simulink model "FeedbackLin"  (R2016a)
settings: Solver=ode45  StartTime=0.0  StopTime=2*Tpasso  FixedStep=1e-4  RelTol=1e-5
values from neighbouring files (symbols this model uses):
  Bm = 1e-4    (= 0.0001)    [runTests.m]
  cm = [c1; c2; c3; c4; c5]    [runTests.m]
  Cphi = 1    [runTests.m]
  cr = [c1; c2; c3; c4; c5]    [runTests.m]
  dQ0 = [dQ10; dQ20; dQ30; dQ40; dQ50]    [runNoErrorNoNoiseNoIncNoFext.m]    (also in runTests.m = zeros(5,1))
  gait = 1    [runTests.m]
  gm = g    (= 9.81)    [runTests.m]
  gr = g    (= 9.81)    [runTests.m]
  Im = [I1; I2; I3; I4; I5]    [runTests.m]
  Ir = [I1; I2; I3; I4; I5]    [runTests.m]
  Jm = 5e-3    (= 0.005)    [runTests.m]
  Kt = 0.1    [runTests.m]
  La = 1e-3    (= 0.001)    [runTests.m]
  LambdaFL = [150; 150; 150; 150]    [runTests.m]
  lm = [l1; l2; l3; l4; l5]    [runTests.m]
  lr = [l1; l2; l3; l4; l5]    [runTests.m]
  mInc = tan(Inc*pi/180)    [runTests.m]
  mm = [m1; m2; m3; m4; m5]    [runTests.m]
  mr = [m1; m2; m3; m4; m5]    [runTests.m]
  pertAmp = 0    [runTests.m]
  pertDur = 0    [runTests.m]
  pertStep = 0    [runTests.m]
  Q0 = [Q10; Q20; Q30; Q40; Q50]    [runNoErrorNoNoiseNoIncNoFext.m]    (also in runTests.m = [pi/2 - pi/10; pi/5; 2*pi-pi/10; pi+pi/10; -pi/4.5])
  Ra = 1    [runTests.m]
  Tpasso = 0.35    [runTests.m]
  TsC = 0.003    [runTests.m]
  TsPID = 1/1000    (= 0.001)    [runTests.m]
  useNoise = false    [runTests.m]
undefined symbols (not defined in the file or in its folder): curStep, Rp1, Rp2
libraries: simulink x8, commrandsrc3 x2
(part 3 of 3)

== matlab function FeedbackLin/getDesiredCoords/High Level Controller - Bézier (FL) ==
  data: dQ input; Q input; Yd output; t input; dYd output; ddYd output; Tpasso parameter; lm parameter; mm parameter; gm parameter; rCPend output; cm parameter; Q0 parameter; dQ0 parameter; ZCoM output; dXCoM output; dxsw0 output; dysw0 output; XCoM output; rCP0 output; curStep parameter
function [Yd, dYd, ddYd, rCPend,  ZCoM, dXCoM, dxsw0, dysw0, XCoM, rCP0]= HighLevel(dQ, Q, t, Tpasso, lm, mm, gm, cm, Q0, dQ0, curStep)
    %Rstep should be calculated from the capture point. Rember here that
    %the total length of the step is divided half before the stance feet
    %(origin of the system) and half after the stance feet. So the Rstep
    %should be twice the desired step position that comes from the capture
    %point. We will calculate de prediction of the capture point at the end
    %of the step and gradually update our Rstep to its value.
    
    %References
%     distCP = 0.0022;     %To have exactly the same step size as the SMC with 0.005
    distCP = 0.005;    %To have the same distCP as the SMC
%     distCP = 0.01 + floor(min(curStep, 49)/5)*0.0025/2; %Was used just to find Lmax
    
    Taux   = Tpasso;    %Seconds. Aux = Trunk oscillation

    Aaux   = 0;         %The trunk inclination is defined as a constant plus a
    phiaux = 0;         %sine according to the following equation:
    aux0   = 0*pi/180;   %aux0 + Aaux*sin(waux*T + phiaux), in rads.
    Yrefh  = 0.29;       %Height to be maintained by the CoM.
    
    Rstep = 0.2;
    
    waux = 2*pi/Taux;
    feetH = 0.01;
    
    %Parameters
    c1 = cm(1);
    c2 = cm(2);
    c3 = cm(3);
    c4 = cm(4);
    c5 = cm(5);
    
    l1 = lm(1);
    l2 = lm(2);
    l3 = lm(3);
    l4 = lm(4);
    l5 = lm(5);
    
    m1 = mm(1);
    m2 = mm(2);
    m3 = mm(3);
    m4 = mm(4);
    m5 = mm(5);
    
    %Position and velocities
    q1 = Q(1);
    q2 = Q(2);
    q3 = Q(3);
    q4 = Q(4);
    q5 = Q(5);
    
    dq1 = dQ(1);
    dq2 = dQ(2);
    dq3 = dQ(3);
    dq4 = dQ(4);
    dq5 = dQ(5);
    
    %Initial Position and velocities
    q10 = Q0(1);
    q20 = Q0(2);
    q30 = Q0(3);
    q40 = Q0(4);
    q50 = Q0(5);
    
    dq10 = dQ0(1);
    dq20 = dQ0(2);
    dq30 = dQ0(3);
    dq40 = dQ0(4);
    dq50 = dQ0(5);
    
    %Important positions for the CoM
    O = [0, 0];
    
    A  = O + l1*[cos(q1), sin(q1)];
    B  = A + l2*[cos(q1+q2), sin(q1+q2)];
    C  = B + l4*[cos(q1+q2+q3+q4), sin(q1+q2+q3+q4)];

    P1 = O + (l1-c1)*[cos(q1), sin(q1)];
    P2 = A + (l2-c2)*[cos(q1+q2), sin(q1+q2)];
    P3 = B + c3*[cos(q1+q2+q3), sin(q1+q2+q3)];
    P4 = B + c4*[cos(q1+q2+q3+q4), sin(q1+q2+q3+q4)];
    P5 = C + c5*[cos(q1+q2+q3+q4+q5), sin(q1+q2+q3+q4+q5)];

    ZCoM = (m1*P1(2) + m2*P2(2) + m3*P3(2) + m4*P4(2) + m5*P5(2))/(m1+m2+m3+m4+m5);
    XCoM = (m1*P1(1) + m2*P2(1) + m3*P3(1) + m4*P4(1) + m5*P5(1))/(m1+m2+m3+m4+m5);
    
    VP1x = -dq1*(l1 - c1)*sin(q1);
    VP2x = -dq1*((l2 - c2)*sin(q1 + q2) + l1*sin(q1)) - dq2*(l2 - c2)*sin(q1 + q2);
    VP3x = -dq1*(l2*sin(q1 + q2) + l1*sin(q1) + c3*sin(q1 + q2 + q3)) - dq2*(l2*sin(q1 + q2) + c3*sin(q1 + q2 + q3)) - c3*dq3*sin(q1 + q2 + q3);
    VP4x = -dq1*(c4*sin(q1 + q2 + q3 + q4) + l2*sin(q1 + q2) + l1*sin(q1)) - dq2*(c4*sin(q1 + q2 + q3 + q4) + l2*sin(q1 + q2)) - c4*dq3*sin(q1 + q2 + q3 + q4) - c4*dq4*sin(q1 + q2 + q3 + q4);
    VP5x = -dq3*(l4*sin(q1 + q2 + q3 + q4) + c5*sin(q1 + q2 + q3 + q4 + q5)) - dq4*(l4*sin(q1 + q2 + q3 + q4) + c5*sin(q1 + q2 + q3 + q4 + q5)) - dq1*(l4*sin(q1 + q2 + q3 + q4) + l2*sin(q1 + q2) + l1*sin(q1) + c5*sin(q1 + q2 + q3 + q4 + q5)) - dq2*(l4*sin(q1 + q2 + q3 + q4) + l2*sin(q1 + q2) + c5*sin(q1 + q2 + q3 + q4 + q5)) - c5*dq5*sin(q1 + q2 + q3 + q4 + q5);
    
    dXCoM = (m1*VP1x + m2*VP2x + m3*VP3x + m4*VP4x + m5*VP5x)/(m1+m2+m3+m4+m5);
    
    %Computation of the current capture point and the capture point
    %expected at the end of the step
    rCP0   = XCoM + dXCoM*sqrt(ZCoM/gm);
    if(Tpasso > t)
        rCPend = rCP0*exp(Tpasso-t);
    else
        rCPend = rCP0;
    end
    
    %Auxiliar - Initial positions and speeds
    O = [0, 0];

    A0  = O  + l1*[cos(q10), sin(q10)];
    B0  = A0 + l2*[cos(q10+q20), sin(q10+q20)];
    C0  = B0 + l4*[cos(q10+q20+q30+q40), sin(q10+q20+q30+q40)];

    P10 = O + (l1-c1)*[cos(q10), sin(q10)];
    P20 = A0 + (l2-c2)*[cos(q10+q20), sin(q10+q20)];
    P30 = B0 + c3*[cos(q10+q20+q30), sin(q10+q20+q30)];
    P40 = B0 + c4*[cos(q10+q20+q30+q40), sin(q10+q20+q30+q40)];
    P50 = C0 + c5*[cos(q10+q20+q30+q40+q50), sin(q10+q20+q30+q40+q50)];
    
    VP10 = [ dq10*sin(q10)*(c1 - l1), -dq10*cos(q10)*(c1 - l1)];
    VP20 = [ dq10*(sin(q10 + q20)*(c2 - l2) - l1*sin(q10)) + dq20*sin(q10 + q20)*(c2 - l2), - dq10*(cos(q10 + q20)*(c2 - l2) - l1*cos(q10)) - dq20*cos(q10 + q20)*(c2 - l2)];
    VP30 = [-dq10*(l2*sin(q10 + q20) + l1*sin(q10) + c3*sin(q10 + q20 + q30)) - dq20*(l2*sin(q10 + q20) + c3*sin(q10 + q20 + q30)) - c3*dq30*sin(q10 + q20 + q30), dq10*(l2*cos(q10 + q20) + l1*cos(q10) + c3*cos(q10 + q20 + q30)) + dq20*(l2*cos(q10 + q20) + c3*cos(q10 + q20 + q30)) + c3*dq30*cos(q10 + q20 + q30)];
    VP40 = [-dq10*(c4*sin(q10 + q20 + q30 + q40) + l2*sin(q10 + q20) + l1*sin(q10)) - dq20*(c4*sin(q10 + q20 + q30 + q40) + l2*sin(q10 + q20)) - c4*dq30*sin(q10 + q20 + q30 + q40) - c4*dq40*sin(q10 + q20 + q30 + q40), dq10*(c4*cos(q10 + q20 + q30 + q40) + l2*cos(q10 + q20) + l1*cos(q10)) + dq20*(c4*cos(q10 + q20 + q30 + q40) + l2*cos(q10 + q20)) + c4*dq30*cos(q10 + q20 + q30 + q40) + c4*dq40*cos(q10 + q20 + q30 + q40)];
    VP50 = [-dq30*(l4*sin(q10 + q20 + q30 + q40) + c5*sin(q10 + q20 + q30 + q40 + q50)) - dq40*(l4*sin(q10 + q20 + q30 + q40) + c5*sin(q10 + q20 + q30 + q40 + q50)) - dq10*(l4*sin(q10 + q20 + q30 + q40) + l2*sin(q10 + q20) + l1*sin(q10) + c5*sin(q10 + q20 + q30 + q40 + q50)) - dq20*(l4*sin(q10 + q20 + q30 + q40) + l2*sin(q10 + q20) + c5*sin(q10 + q20 + q30 + q40 + q50)) - c5*dq50*sin(q10 + q20 + q30 + q40 + q50), dq30*(l4*cos(q10 + q20 + q30 + q40) + c5*cos(q10 + q20 + q30 + q40 + q50)) + dq40*(l4*cos(q10 + q20 + q30 + q40) + c5*cos(q10 + q20 + q30 + q40 + q50)) + dq10*(l4*cos(q10 + q20 + q30 + q40) + l2*cos(q10 + q20) + l1*cos(q10) + c5*cos(q10 + q20 + q30 + q40 + q50)) + dq20*(l4*cos(q10 + q20 + q30 + q40) + l2*cos(q10 + q20) + c5*cos(q10 + q20 + q30 + q40 + q50)) + c5*dq50*cos(q10 + q20 + q30 + q40 + q50)];
    
    xsw0  = l1*cos(q10) + l2*cos(q10+q20) + l4*cos(q10+q20+q30+q40) + l5*cos(q10+q20+q30+q40+q50);
    ysw0  = l1*sin(q10) + l2*sin(q10+q20) + l4*sin(q10+q20+q30+q40) + l5*sin(q10+q20+q30+q40+q50);
    qt0   = (5*pi/2) - q10 - q20 - q30;
    ycom0 = (m1*P10(2) + m2*P20(2) + m3*P30(2) + m4*P40(2) + m5*P50(2))/(m1+m2+m3+m4+m5);
    
    dxsw0  = -l1*sin(q10)*dq10 - l2*sin(q10+q20)*(dq10+dq20) - l4*sin(q10+q20+q30+q40)*(dq10+dq20+dq30+dq40) - l5*sin(q10+q20+q30+q40+q50)*(dq10+dq20+dq30+dq40+dq50);
    dysw0  = +l1*cos(q10)*dq10 + l2*cos(q10+q20)*(dq10+dq20) + l4*cos(q10+q20+q30+q40)*(dq10+dq20+dq30+dq40) + l5*cos(q10+q20+q30+q40+q50)*(dq10+dq20+dq30+dq40+dq50);
    dqt0   = -dq10 - dq20 - dq30;
    dycom0 = (m1*VP10(2) + m2*VP20(2) + m3*VP30(2) + m4*VP40(2) + m5*VP50(2))/(m1+m2+m3+m4+m5);
    
    %Bézier
    
    %Xsw
    DF = rCPend - distCP;
%     if(DF > 0.1688)
%         DF = 0.1688;
%     end
%     DF = Rstep/2;

    b0xsw0 = xsw0;
    b1xsw0 = b0xsw0 + dxsw0*Tpasso*(1/7);
    b2xsw0 = b1xsw0 + (DF - b1xsw0)*3/5;
    b3xsw0 = b1xsw0 + (DF - b1xsw0)*4/5;
    b4xsw0 = DF;
    b5xsw0 = DF;
    b6xsw0 = DF;
    b7xsw0 = DF;
    
    %Ysw
    b0ysw0 = ysw0;
    b1ysw0 = b0ysw0 + dysw0*Tpasso/7;
    b2ysw0 = feetH;
    b3ysw0 = feetH;
    b4ysw0 = feetH;
    b5ysw0 = feetH;
    b6ysw0 = feetH;
    b7ysw0 = -feetH/2;
    
    %qt
    b0qt0 = qt0;
    b1qt0 = b0qt0 + dqt0*Tpasso/7;
    b2qt0 = b1qt0 + (aux0-b1qt0)*1/4;
    b3qt0 = b1qt0 + (aux0-b1qt0)*2/4;
    b4qt0 = b1qt0 + (aux0-b1qt0)*3/4;
    b5qt0 = aux0;
    b6qt0 = aux0;
    b7qt0 = aux0;
    
    %yCoM
    b0ycom0 = ycom0;
    b1ycom0 = b0ycom0 + dycom0*Tpasso/7;
    b2ycom0 = b1ycom0 + (Yrefh-b1ycom0)*1/4;
    b3ycom0 = b1ycom0 + (Yrefh-b1ycom0)*2/4;
    b4ycom0 = b1ycom0 + (Yrefh-b1ycom0)*3/4;
    b5ycom0 = Yrefh;
    b6ycom0 = Yrefh;
    b7ycom0 = Yrefh;
    
    taux = t/Tpasso;
    
    %% Casteljau's Algorithm
    %xsw
    b0xsw1 = (1 - taux)*b0xsw0 + taux*b1xsw0;
    b1xsw1 = (1 - taux)*b1xsw0 + taux*b2xsw0;
    b2xsw1 = (1 - taux)*b2xsw0 + taux*b3xsw0;
    b3xsw1 = (1 - taux)*b3xsw0 + taux*b4xsw0;
    b4xsw1 = (1 - taux)*b4xsw0 + taux*b5xsw0;
    b5xsw1 = (1 - taux)*b5xsw0 + taux*b6xsw0;
    b6xsw1 = (1 - taux)*b6xsw0 + taux*b7xsw0;
    
    b0xsw2 = (1 - taux)*b0xsw1 + taux*b1xsw1;
    b1xsw2 = (1 - taux)*b1xsw1 + taux*b2xsw1;
    b2xsw2 = (1 - taux)*b2xsw1 + taux*b3xsw1;
    b3xsw2 = (1 - taux)*b3xsw1 + taux*b4xsw1;
    b4xsw2 = (1 - taux)*b4xsw1 + taux*b5xsw1;
    b5xsw2 = (1 - taux)*b5xsw1 + taux*b6xsw1;
  
    b0xsw3 = (1 - taux)*b0xsw2 + taux*b1xsw2;
    b1xsw3 = (1 - taux)*b1xsw2 + taux*b2xsw2;
    b2xsw3 = (1 - taux)*b2xsw2 + taux*b3xsw2;
    b3xsw3 = (1 - taux)*b3xsw2 + taux*b4xsw2;
    b4xsw3 = (1 - taux)*b4xsw2 + taux*b5xsw2;
    
    b0xsw4 = (1 - taux)*b0xsw3 + taux*b1xsw3;
    b1xsw4 = (1 - taux)*b1xsw3 + taux*b2xsw3;
    b2xsw4 = (1 - taux)*b2xsw3 + taux*b3xsw3;
    b3xsw4 = (1 - taux)*b3xsw3 + taux*b4xsw3;
   
    b0xsw5 = (1 - taux)*b0xsw4 + taux*b1xsw4;
    b1xsw5 = (1 - taux)*b1xsw4 + taux*b2xsw4;
    b2xsw5 = (1 - taux)*b2xsw4 + taux*b3xsw4;
    
    b0xsw6 = (1 - taux)*b0xsw5 + taux*b1xsw5;
    b1xsw6 = (1 - taux)*b1xsw5 + taux*b2xsw5;
   
    b0xsw7 = (1 - taux)*b0xsw6 + taux*b1xsw6;
    
    %ysw
    b0ysw1 = (1 - taux)*b0ysw0 + taux*b1ysw0;
    b1ysw1 = (1 - taux)*b1ysw0 + taux*b2ysw0;
    b2ysw1 = (1 - taux)*b2ysw0 + taux*b3ysw0;
    b3ysw1 = (1 - taux)*b3ysw0 + taux*b4ysw0;
    b4ysw1 = (1 - taux)*b4ysw0 + taux*b5ysw0;
    b5ysw1 = (1 - taux)*b5ysw0 + taux*b6ysw0;
    b6ysw1 = (1 - taux)*b6ysw0 + taux*b7ysw0;
    
    b0ysw2 = (1 - taux)*b0ysw1 + taux*b1ysw1;
    b1ysw2 = (1 - taux)*b1ysw1 + taux*b2ysw1;
    b2ysw2 = (1 - taux)*b2ysw1 + taux*b3ysw1;
    b3ysw2 = (1 - taux)*b3ysw1 + taux*b4ysw1;
    b4ysw2 = (1 - taux)*b4ysw1 + taux*b5ysw1;
    b5ysw2 = (1 - taux)*b5ysw1 + taux*b6ysw1;
  
    b0ysw3 = (1 - taux)*b0ysw2 + taux*b1ysw2;
    b1ysw3 = (1 - taux)*b1ysw2 + taux*b2ysw2;
    b2ysw3 = (1 - taux)*b2ysw2 + taux*b3ysw2;
    b3ysw3 = (1 - taux)*b3ysw2 + taux*b4ysw2;
    b4ysw3 = (1 - taux)*b4ysw2 + taux*b5ysw2;
    
    b0ysw4 = (1 - taux)*b0ysw3 + taux*b1ysw3;
    b1ysw4 = (1 - taux)*b1ysw3 + taux*b2ysw3;
    b2ysw4 = (1 - taux)*b2ysw3 + taux*b3ysw3;
    b3ysw4 = (1 - taux)*b3ysw3 + taux*b4ysw3;
   
    b0ysw5 = (1 - taux)*b0ysw4 + taux*b1ysw4;
    b1ysw5 = (1 - taux)*b1ysw4 + taux*b2ysw4;
    b2ysw5 = (1 - taux)*b2ysw4 + taux*b3ysw4;
    
    b0ysw6 = (1 - taux)*b0ysw5 + taux*b1ysw5;
    b1ysw6 = (1 - taux)*b1ysw5 + taux*b2ysw5;
   
    b0ysw7 = (1 - taux)*b0ysw6 + taux*b1ysw6;
    
    %Qt
    b0qt1 = (1 - taux)*b0qt0 + taux*b1qt0;
    b1qt1 = (1 - taux)*b1qt0 + taux*b2qt0;
    b2qt1 = (1 - taux)*b2qt0 + taux*b3qt0;
    b3qt1 = (1 - taux)*b3qt0 + taux*b4qt0;
    b4qt1 = (1 - taux)*b4qt0 + taux*b5qt0;
    b5qt1 = (1 - taux)*b5qt0 + taux*b6qt0;
    b6qt1 = (1 - taux)*b6qt0 + taux*b7qt0;
    
    b0qt2 = (1 - taux)*b0qt1 + taux*b1qt1;
    b1qt2 = (1 - taux)*b1qt1 + taux*b2qt1;
    b2qt2 = (1 - taux)*b2qt1 + taux*b3qt1;
    b3qt2 = (1 - taux)*b3qt1 + taux*b4qt1;
    b4qt2 = (1 - taux)*b4qt1 + taux*b5qt1;
    b5qt2 = (1 - taux)*b5qt1 + taux*b6qt1;
    
    b0qt3 = (1 - taux)*b0qt2 + taux*b1qt2;
    b1qt3 = (1 - taux)*b1qt2 + taux*b2qt2;
    b2qt3 = (1 - taux)*b2qt2 + taux*b3qt2;
    b3qt3 = (1 - taux)*b3qt2 + taux*b4qt2;
    b4qt3 = (1 - taux)*b4qt2 + taux*b5qt2;
    
    b0qt4 = (1 - taux)*b0qt3 + taux*b1qt3;
    b1qt4 = (1 - taux)*b1qt3 + taux*b2qt3;
    b2qt4 = (1 - taux)*b2qt3 + taux*b3qt3;
    b3qt4 = (1 - taux)*b3qt3 + taux*b4qt3;
   
    b0qt5 = (1 - taux)*b0qt4 + taux*b1qt4;
    b1qt5 = (1 - taux)*b1qt4 + taux*b2qt4;
    b2qt5 = (1 - taux)*b2qt4 + taux*b3qt4;
    
    b0qt6 = (1 - taux)*b0qt5 + taux*b1qt5;
    b1qt6 = (1 - taux)*b1qt5 + taux*b2qt5;
   
    b0qt7 = (1 - taux)*b0qt6 + taux*b1qt6;
    
    %yCoM
    b0ycom1 = (1 - taux)*b0ycom0 + taux*b1ycom0;
    b1ycom1 = (1 - taux)*b1ycom0 + taux*b2ycom0;
    b2ycom1 = (1 - taux)*b2ycom0 + taux*b3ycom0;
    b3ycom1 = (1 - taux)*b3ycom0 + taux*b4ycom0;
    b4ycom1 = (1 - taux)*b4ycom0 + taux*b5ycom0;
    b5ycom1 = (1 - taux)*b5ycom0 + taux*b6ycom0;
    b6ycom1 = (1 - taux)*b6ycom0 + taux*b7ycom0;
    
    b0ycom2 = (1 - taux)*b0ycom1 + taux*b1ycom1;
    b1ycom2 = (1 - taux)*b1ycom1 + taux*b2ycom1;
    b2ycom2 = (1 - taux)*b2ycom1 + taux*b3ycom1;
    b3ycom2 = (1 - taux)*b3ycom1 + taux*b4ycom1;
    b4ycom2 = (1 - taux)*b4ycom1 + taux*b5ycom1;
    b5ycom2 = (1 - taux)*b5ycom1 + taux*b6ycom1;
    
    b0ycom3 = (1 - taux)*b0ycom2 + taux*b1ycom2;
    b1ycom3 = (1 - taux)*b1ycom2 + taux*b2ycom2;
    b2ycom3 = (1 - taux)*b2ycom2 + taux*b3ycom2;
    b3ycom3 = (1 - taux)*b3ycom2 + taux*b4ycom2;
    b4ycom3 = (1 - taux)*b4ycom2 + taux*b5ycom2;
    
    b0ycom4 = (1 - taux)*b0ycom3 + taux*b1ycom3;
    b1ycom4 = (1 - taux)*b1ycom3 + taux*b2ycom3;
    b2ycom4 = (1 - taux)*b2ycom3 + taux*b3ycom3;
    b3ycom4 = (1 - taux)*b3ycom3 + taux*b4ycom3;
   
    b0ycom5 = (1 - taux)*b0ycom4 + taux*b1ycom4;
    b1ycom5 = (1 - taux)*b1ycom4 + taux*b2ycom4;
    b2ycom5 = (1 - taux)*b2ycom4 + taux*b3ycom4;
    
    b0ycom6 = (1 - taux)*b0ycom5 + taux*b1ycom5;
    b1ycom6 = (1 - taux)*b1ycom5 + taux*b2ycom5;
   
    b0ycom7 = (1 - taux)*b0ycom6 + taux*b1ycom6;
    
    %Resulting system
    xsw  = b0xsw7;
    ysw  = b0ysw7;
    qt2   = b0qt7;
    yCoM2 = b0ycom7;
    
    dxsw  = 7*(b1xsw6  - b0xsw6)/Tpasso;
    dysw  = 7*(b1ysw6  - b0ysw6)/Tpasso;
    dqt2   = 7*(b1qt6   - b0qt6)/Tpasso;
    dyCoM2 = 7*(b1ycom6 - b0ycom6)/Tpasso;
    
    ddxsw  = 7*6*(b2xsw5  - 2*b1xsw5  + b0xsw5)/(Tpasso^2);
    ddysw  = 7*6*(b2ysw5  - 2*b1ysw5  + b0ysw5)/(Tpasso^2);
    ddqt2   = 7*6*(b2qt5   - 2*b1qt5   + b0qt5)/(Tpasso^2);
    ddyCoM2 = 7*6*(b2ycom5 - 2*b1ycom5 + b0ycom5)/(Tpasso^2);
    
    
    yCoM = Yrefh;
    qt = aux0 + Aaux*sin(waux*t + phiaux);
    
    dyCoM = 0;
    dqt = Aaux*waux*cos(waux*t + phiaux);
    
    ddyCoM = 0;
    ddqt = -Aaux*waux^2*sin(waux*t + phiaux);
   
    
    Yd   = [  qt2;   ysw;   yCoM2;   xsw];
    dYd  = [ dqt2;  dysw;  dyCoM2;  dxsw];
    ddYd = [ddqt2; ddysw; ddyCoM2; ddxsw];
end
